simulink model "Sparus_3D_advance_model"  (R2021b)
settings: Solver=ode3  StartTime=0.0  StopTime=200  FixedStep=0.01  RelTol=1e-3  EnableMultiTasking=on
InitFcn:
  | Para=Parameters()
StopFcn:
  | Plotting
undefined symbols (not defined in the file or in its folder): Command, MeaSim, RovModel
settings Model: Creator=Thomas  LastModifiedBy=Eduardo
settings SolverCC: AlgebraicLoopSolver=TrustRegion
settings DataIOCC: LimitDataPoints=on  SaveFormat=Array  SignalLoggingSaveFormat=ModelDataLogs  ReturnWorkspaceOutputs=off
settings OptimizationCC: ExpressionDepthLimit=2147483647  LifeSpan=inf
settings DebuggingCC: UnderspecifiedInitializationDetection=Classic  MergeDetectMultiDrivingBlocksExec=none  SolverPrmCheckMsg=warning  FcnCallInpInsideContextMsg=warning  StateNameClashWarn=warning  SFUnexpectedBacktrackingDiag=warning  SFNoUnconditionalDefaultTransitionDiag=warning  SFExecutionAtInitializationDiag=none  SFMachineParentedDataDiag=warning  ArithmeticOperatorsInVariantConditions=warning
settings HardwareCC: ProdBitPerPointer=32  ProdBitPerSizeT=32  ProdBitPerPtrDiffT=32  ProdLargestAtomicFloat=None  ProdIntDivRoundTo=Undefined  ProdEndianess=Unspecified  ProdWordSize=32  ProdHWDeviceType=32-bit Generic
settings ModelReferenceCC: PropagateSignalLabelsOutOfModel=off
settings SFSimCC: SimUseLocalCustomCode=off  SimParseCustomCode=off  SimGenImportedTypeDefs=on  CustomCodeUndefinedFunction=UseInterfaceOnly  SimTargetLang=C++
settings RTWCC: Description="Create Visual C/C++ Solution File for the \"grt\" target"  GenCodeOnly=on  TemplateMakefile=RTW.MSVCBuild  RTWUseLocalCustomCode=off  TargetLang=C++
settings CodeAppCC: StateflowObjectComments=on
settings GRTTargetCC: TargetLangStandard=C89/C90 (ANSI)  CombineOutputUpdateFcns=off  GRTInterface=on
settings ConfigComp: CovMetricSettings=dw  CovSaveCumulativeToWorkspaceVar=on  CovSaveSingleToWorkspaceVar=on  CovExternalEMLEnable=off  CovSFcnEnable=off

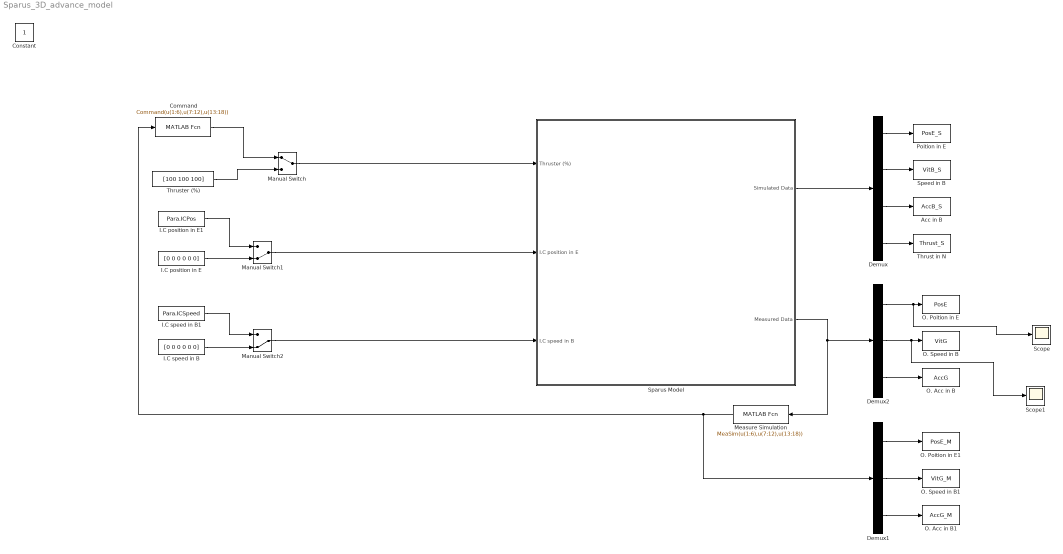
== system Sparus_3D_advance_model ==
  Acc in B : ToWorkspace  VariableName=AccB_S  SampleTime=-1
  Command : MATLABFcn  MATLABFcn=Command(u(1:6),u(7:12),u(13:18))  OutputDimensions=3  OutputSignalType=real
  Demux : Demux  Outputs=[6 6 6 3]
  Demux1 : Demux  Outputs=3
  Demux2 : Demux  Outputs=[6 6 6]
  I.C position in E : Constant  Value=[0 0 0 0 0 0]
  I.C position in E1 : Constant  Value=Para.ICPos
  I.C speed in B : Constant  Value=[0 0 0 0 0 0]
  I.C speed in B1 : Constant  Value=Para.ICSpeed
  Manual Switch : ManualSwitch
  Manual Switch1 : ManualSwitch  CurrentSetting=0
  Manual Switch2 : ManualSwitch  CurrentSetting=0
  Measure Simulation : MATLABFcn  MATLABFcn=MeaSim(u(1:6),u(7:12),u(13:18))  OutputDimensions=18  OutputSignalType=real
  O. Acc in B : ToWorkspace  VariableName=AccG  SampleTime=-1
  O. Acc in B1 : ToWorkspace  VariableName=AccG_M  SampleTime=-1
  O. Poition in E : ToWorkspace  VariableName=PosE  SampleTime=-1
  O. Poition in E1 : ToWorkspace  VariableName=PosE_M  SampleTime=-1
  O. Speed in B : ToWorkspace  VariableName=VitG  SampleTime=-1
  O. Speed in B1 : ToWorkspace  VariableName=VitG_M  SampleTime=-1
  Poition in E : ToWorkspace  VariableName=PosE_S  SampleTime=-1
  Scope : Scope
  Scope1 : Scope
  Sparus Model : Subsystem
  Speed in B : ToWorkspace  VariableName=VitB_S  SampleTime=-1
  Thrust in N : ToWorkspace  VariableName=Thrust_S  SampleTime=-1
  Thruster (%) : Constant  Value=[100 100 100]
  Constant : Constant  IOType=siggen
  wires:
  Manual Switch/1 -> Sparus Model/1(Thruster (%))
  Demux/4 -> Thrust in N/1
  Demux/3 -> Acc in B/1
  Demux/2 -> Speed in B/1
  Demux/1 -> Poition in E/1
  Sparus Model/1(Simulated Data) -> Demux/1
  Sparus Model/2("Measured Data ") -> Measure Simulation/1, Demux2/1
  Thruster (%)/1 -> Manual Switch/2
  Command/1 -> Manual Switch/1
  I.C position in E1/1 -> Manual Switch1/1
  I.C speed in B1/1 -> Manual Switch2/1
  Manual Switch2/1 -> Sparus Model/3("I.C speed in B ")
  I.C speed in B/1 -> Manual Switch2/2
  Manual Switch1/1 -> Sparus Model/2(I.C position in E)
  I.C position in E/1 -> Manual Switch1/2
  Demux2/3 -> O. Acc in B/1
  Demux2/2 -> Scope1/1, O. Speed in B/1
  Demux2/1 -> Scope/1, O. Poition in E/1
  Measure Simulation/1 -> Demux1/1, Command/1
  Demux1/3 -> O. Acc in B1/1
  Demux1/2 -> O. Speed in B1/1
  Demux1/1 -> O. Poition in E1/1

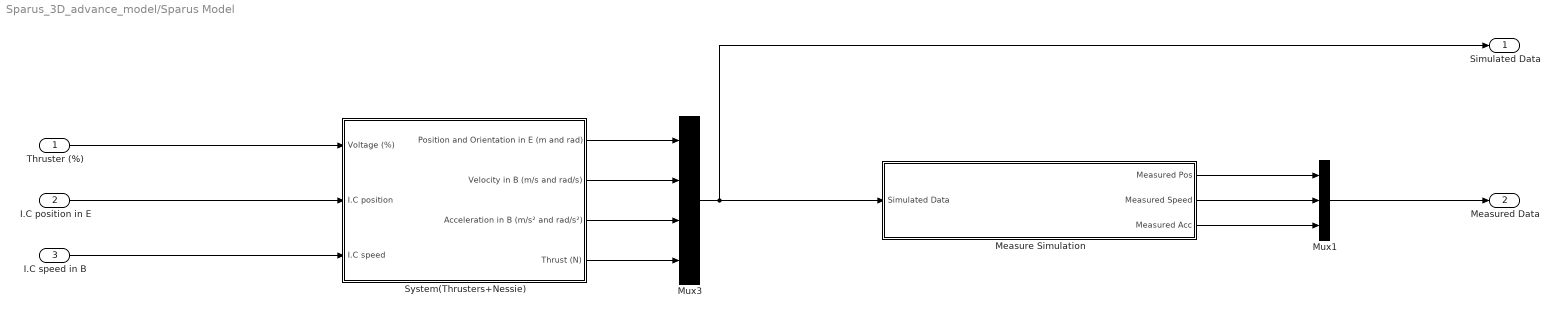
== system Sparus_3D_advance_model/Sparus Model ==
  Thruster (%) : Inport
  I.C position in E : Inport  Port=2
  "I.C speed in B " : Inport  Port=3
  Measure Simulation : Subsystem
  Mux1 : Mux  Inputs=3
  Mux3 : Mux
  System(Thrusters+Nessie) : Subsystem
  Simulated Data : Outport
  "Measured Data " : Outport  Port=2
  wires:
  I.C position in E/1 -> System(Thrusters+Nessie)/2(I.C position)
  System(Thrusters+Nessie)/3(Acceleration in B (m/s² and rad/s²)) -> Mux3/3
  Thruster (%)/1 -> System(Thrusters+Nessie)/1(Voltage (%))
  Mux1/1 -> "Measured Data "/1
  System(Thrusters+Nessie)/1(Position and Orientation in E (m and rad)) -> Mux3/1
  "I.C speed in B "/1 -> System(Thrusters+Nessie)/3(I.C speed)
  System(Thrusters+Nessie)/2(Velocity in B (m/s and rad/s)) -> Mux3/2
  System(Thrusters+Nessie)/4(Thrust (N)) -> Mux3/4
  Mux3/1 -> Simulated Data/1, Measure Simulation/1("Simulated Data ")
  Measure Simulation/1(Measured Pos) -> Mux1/1
  Measure Simulation/2(Measured Speed) -> Mux1/2
  Measure Simulation/3(Measured Acc) -> Mux1/3

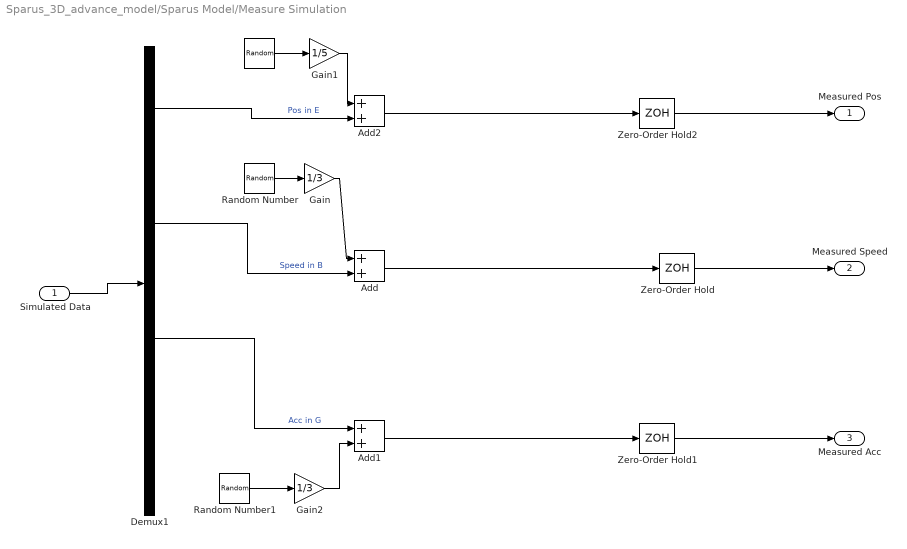
== system Sparus_3D_advance_model/Sparus Model/Measure Simulation ==
  "Simulated Data " : Inport
  " " : RandomNumber  Variance=0.01
  Add : Sum
  Add1 : Sum
  Add2 : Sum
  Demux1 : Demux  Outputs=[6 6 6 3]
  Gain : Gain  Gain=1/3
  Gain1 : Gain  Gain=1/5
  Gain2 : Gain  Gain=1/3
  Random Number : RandomNumber  Variance=0.01
  Random Number1 : RandomNumber  Variance=0.1
  Zero-Order Hold : ZeroOrderHold  SampleTime=-1
  Zero-Order Hold1 : ZeroOrderHold  SampleTime=-1
  Zero-Order Hold2 : ZeroOrderHold  SampleTime=-1
  Measured Pos : Outport
  Measured Speed : Outport  Port=2
  Measured Acc : Outport  Port=3
  wires:
  Add/1 -> Zero-Order Hold/1
  "Simulated Data "/1 -> Demux1/1
  Demux1/3 -> Add1/1  "Acc in G"
  Add1/1 -> Zero-Order Hold1/1
  Demux1/2 -> Add/2  "Speed in B"
  Add2/1 -> Zero-Order Hold2/1
  Demux1/1 -> Add2/2  "Pos in E"
  Random Number/1 -> Gain/1
  Gain/1 -> Add/1
  " "/1 -> Gain1/1
  Gain1/1 -> Add2/1
  Random Number1/1 -> Gain2/1
  Gain2/1 -> Add1/2
  Zero-Order Hold2/1 -> Measured Pos/1
  Zero-Order Hold/1 -> Measured Speed/1
  Zero-Order Hold1/1 -> Measured Acc/1

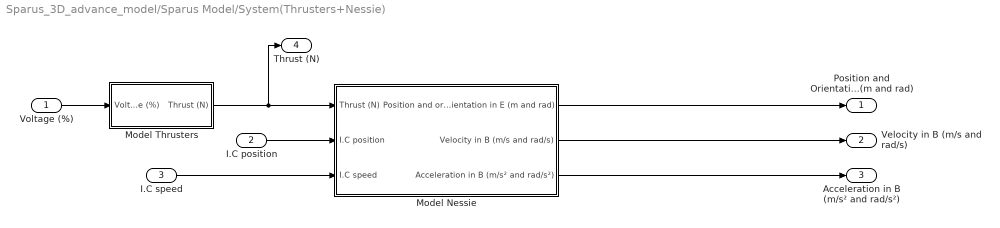
== system Sparus_3D_advance_model/Sparus Model/System(Thrusters+Nessie) ==
  Voltage (%) : Inport
  I.C position : Inport  Port=2
  I.C speed : Inport  Port=3
  Model Nessie : Subsystem
  Model Thrusters : Subsystem
  Position and Orientation in E (m and rad) : Outport
  Velocity in B (m/s and rad/s) : Outport  Port=2
  Acceleration in B (m/s² and rad/s²) : Outport  Port=3
  Thrust (N) : Outport  Port=4
  wires:
  Model Nessie/1(Position and orientation in E (m and rad)) -> Position and Orientation in E (m and rad)/1
  I.C position/1 -> Model Nessie/2(I.C position)
  Model Nessie/2(Velocity in B (m/s and rad/s)) -> Velocity in B (m/s and rad/s)/1
  Voltage (%)/1 -> Model Thrusters/1(Voltage (%))
  Model Thrusters/1(Thrust (N)) -> Model Nessie/1(Thrust (N)), Thrust (N)/1
  Model Nessie/3(Acceleration in B (m/s² and rad/s²)) -> Acceleration in B (m/s² and rad/s²)/1
  I.C speed/1 -> Model Nessie/3(I.C speed)

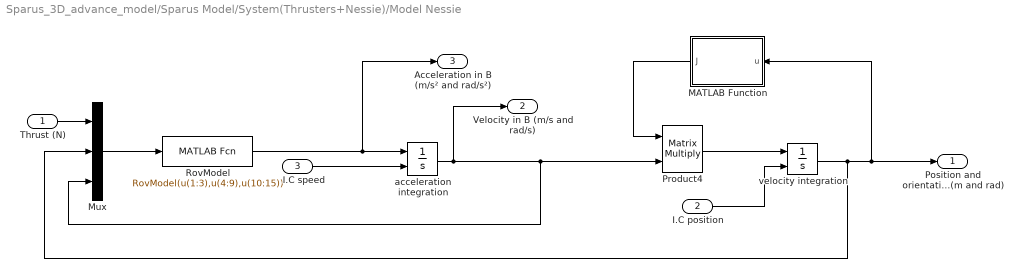
== system Sparus_3D_advance_model/Sparus Model/System(Thrusters+Nessie)/Model Nessie ==
  Thrust (N) : Inport
  I.C position : Inport  Port=2
  I.C speed : Inport  Port=3
  MATLAB Function : MATLAB Function  TreatAsAtomicUnit=on
  Mux : Mux  Inputs=3
  Product4 : Product  Multiplication=Matrix(*)  RndMeth=Zero
  RovModel : MATLABFcn  MATLABFcn=RovModel(u(1:3),u(4:9),u(10:15))  OutputDimensions=6  OutputSignalType=real
  acceleration integration : Integrator  InitialConditionSource=external  InitialCondition=[0 0 0 0 0 0]
  velocity integration : Integrator  InitialConditionSource=external
  Position and orientation in E (m and rad) : Outport
  Velocity in B (m/s and rad/s) : Outport  Port=2
  Acceleration in B (m/s² and rad/s²) : Outport  Port=3
  wires:
  Thrust (N)/1 -> Mux/1
  I.C position/1 -> velocity integration/2
  Product4/1 -> velocity integration/1
  acceleration integration/1 -> Velocity in B (m/s and rad/s)/1, Mux/3, Product4/2
  velocity integration/1 -> MATLAB Function/1(u), Position and orientation in E (m and rad)/1, Mux/2
  RovModel/1 -> acceleration integration/1, Acceleration in B (m/s² and rad/s²)/1
  Mux/1 -> RovModel/1
  I.C speed/1 -> acceleration integration/2
  MATLAB Function/1(J) -> Product4/1

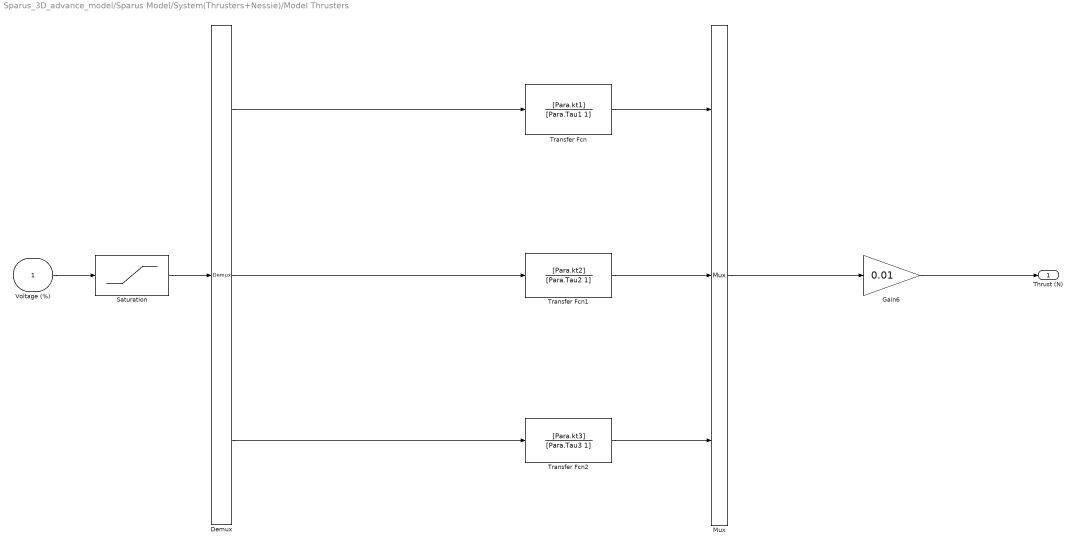
== system Sparus_3D_advance_model/Sparus Model/System(Thrusters+Nessie)/Model Thrusters ==
  Voltage (%) : Inport
  Demux : Demux  Outputs=3
  Gain6 : Gain  Gain=0.01
  Mux : Mux  Inputs=3
  Saturation : Saturate  UpperLimit=100  LowerLimit=-100
  Transfer Fcn : TransferFcn  Numerator=[Para.kt1]  Denominator=[Para.Tau1 1]
  Transfer Fcn1 : TransferFcn  Numerator=[Para.kt2]  Denominator=[Para.Tau2 1]
  Transfer Fcn2 : TransferFcn  Numerator=[Para.kt3]  Denominator=[Para.Tau3 1]
  Thrust (N) : Outport
  wires:
  Mux/1 -> Gain6/1
  Saturation/1 -> Demux/1
  Voltage (%)/1 -> Saturation/1
  Gain6/1 -> Thrust (N)/1
  Transfer Fcn/1 -> Mux/1
  Transfer Fcn1/1 -> Mux/2
  Transfer Fcn2/1 -> Mux/3
  Demux/1 -> Transfer Fcn/1
  Demux/2 -> Transfer Fcn1/1
  Demux/3 -> Transfer Fcn2/1

== matlab function Sparus_3D_advance_model/Sparus Model/System(Thrusters+Nessie)/Model Nessie/MATLAB Function ==
  data: u input; J output
function J = fcn(u)

[~ , ~ , J] = jacobienne(u);

end
